simulink model "formation_control"  (R2021a)
settings: Solver=VariableStepAuto  StartTime=0.0  StopTime=T  RelTol=1e-3
undefined symbols (not defined in the file or in its folder): params
settings Model: Creator=gaeta  LastModifiedBy=18214
settings SolverCC: AlgebraicLoopSolver=TrustRegion
settings DataIOCC: InitialState=initialCondition  LoadInitialState=on
settings DebuggingCC: SFMachineParentedDataDiag=warning

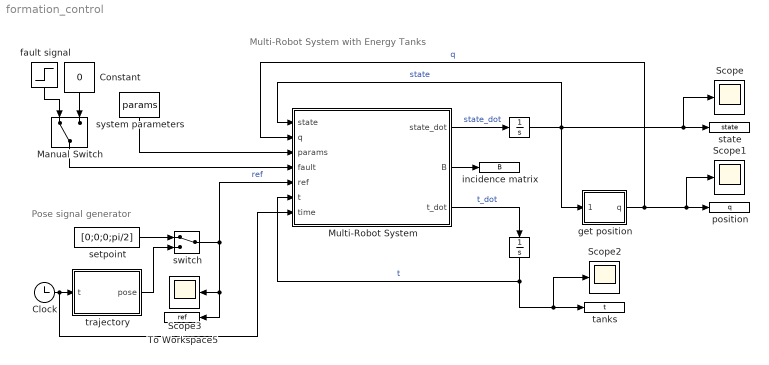
== system formation_control ==
  note: Multi-Robot System with Energy Tanks
  note: Pose signal generator
  "  " : Integrator
  "   " : Integrator
  Clock : Clock
  Constant : Constant  Value=0
  Manual Switch : ManualSwitch
  Multi-Robot System : MATLAB Function  TreatAsAtomicUnit=on
  Scope{,1..3} (4 alike) : Scope
  To Workspace5 : ToWorkspace  VariableName=ref  SaveFormat=Timeseries  SampleTime=-1
  fault signal : Step  Time=25  SampleTime=0
  get position : Subsystem
  incidence matrix : ToWorkspace  VariableName=B  SaveFormat=Timeseries  SampleTime=-1
  position : ToWorkspace  VariableName=q  SaveFormat=Timeseries  SampleTime=-1
  setpoint : Constant  Value=[0;0;0;pi/2]
  state : ToWorkspace  VariableName=state  SaveFormat=Timeseries  SampleTime=-1
  switch : ManualSwitch
  "system parameters " : Constant  Value=params  OutDataTypeStr=Bus: params_bus
  tanks : ToWorkspace  VariableName=t  SaveFormat=Timeseries  SampleTime=-1
  trajectory : MATLAB Function  TreatAsAtomicUnit=on
  wires:
  trajectory/1(pose) -> switch/2
  setpoint/1 -> switch/1
  Clock/1 -> Multi-Robot System/7(time), trajectory/1(t)
  switch/1 -> Multi-Robot System/5(ref), Scope3/1, To Workspace5/1  "ref"
  "system parameters "/1 -> Multi-Robot System/3(params)
  fault signal/1 -> Manual Switch/1
  "  "/1 -> tanks/1, Scope2/1, Multi-Robot System/6(t)  "t"
  Multi-Robot System/1(state_dot) -> "   "/1  "state_dot"
  Multi-Robot System/2(B) -> incidence matrix/1
  "   "/1 -> Multi-Robot System/1(state), Scope/1, state/1, get position/1(state)  "state"
  Multi-Robot System/3(t_dot) -> "  "/1  "t_dot"
  get position/1(q) -> Scope1/1, position/1, Multi-Robot System/2(q)  "q"
  Manual Switch/1 -> Multi-Robot System/4(fault)
  Constant/1 -> Manual Switch/2

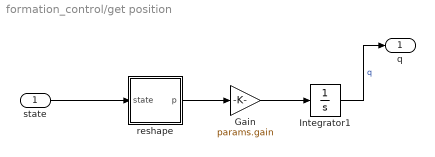
== system formation_control/get position ==
  state : Inport
  Gain : Gain  Gain=params.gain
  Integrator1 : Integrator
  reshape : MATLAB Function  TreatAsAtomicUnit=on
  q : Outport
  wires:
  state/1 -> reshape/1(state)
  reshape/1(p) -> Gain/1
  Gain/1 -> Integrator1/1
  Integrator1/1 -> q/1  "q"

== matlab function formation_control/trajectory ==
  data: pose output size=4; t input size=1
%% 生成参考轨迹
function pose = trajectory(t)
t1 = 5;
t_fault = 25;
t_end = 55;
pause = 5;

w = 0.25;
phi = -w*t1;
A = 80;
z_vel = 1;

y = [0;0;0];
theta = pi/2;
if(t>=t1 && t<t_fault)
    y = [A*sin(w*t+phi); -A*cos(w*t+phi); z_vel*t] - [A*sin(w*t1+phi); -A*cos(w*t1+phi); z_vel*t1];
    theta = atan2(A*sin(w*t+phi), A*cos(w*t+phi));
elseif(t>=t_fault && t<t_fault+pause)
    y = [A*sin(w*t_fault+phi); -A*cos(w*t_fault+phi); z_vel*t_fault] - [A*sin(w*t1+phi); -A*cos(w*t1+phi); z_vel*t1];
    theta = atan2(A*sin(w*t_fault+phi), A*cos(w*t_fault+phi));
elseif(t>=t_fault+pause && t<t_end)
%     y = [A*sin(w*(t-pause)+phi); -A*cos(w*(t-pause)+phi); z_vel*(t-pause)] - [A*sin(w*t1+phi); -A*cos(w*t1+phi); z_vel*t1];
%     theta = atan2(A*sin(w*(t-pause)+phi), A*cos(w*(t-pause)+phi));
    y = [A*sin(w*(t_fault)+phi)+20*w*(t-t_fault-pause); -A*cos(w*(t_fault)+phi)-20*w*(t-t_fault-pause); z_vel*(t_fault)] - [A*sin(w*t1+phi); -A*cos(w*t1+phi); z_vel*t1];
    theta = -pi/4;
elseif(t>=t_end)
%     y = [A*sin(w*(t_end-pause)+phi); -A*cos(w*(t_end-pause)+phi); z_vel*(t_end-pause)] - [A*sin(w*t1+phi); -A*cos(w*t1+phi); z_vel*t1];
%     theta = atan2(A*sin(w*(t_end-pause)+phi), A*cos(w*(t_end-pause)+phi));
    y = [A*sin(w*(t_fault)+phi)+20*w*(t_end-t_fault-pause); -A*cos(w*(t_fault)+phi)-20*w*(t_end-t_fault-pause); z_vel*(t_fault)] - [A*sin(w*t1+phi); -A*cos(w*t1+phi); z_vel*t1];
    theta = -pi/4;
end

pose = [y; theta];
end

== matlab function formation_control/Multi-Robot System ==
  data: state input size=3*(params.N+params.E); q input size=3*params.N; state_dot output size=3*(params.N+params.E); params input; fault input; ref input size=4; t input size=params.N; B output; t_dot output size=params.N; time input
function [state_dot,B,t_dot] = closedLoopSystem(state, q, params, fault, ref, t, time)    % 状态变量（动量、相对位置）、位置、params、失效信号、参考轨迹、能量罐参数（导数）
n = 3;                      % 任务空间
N = params.N;               % Agent数量
faulted_robot = params.faulted_robot;   % 失效Agent

%% 矩阵初始化Ⅰ
p = state(1:n*N);           % Agent动量（状态变量）
m = params.m;               % Agent质量
M = zeros(n*N, n*N);      	% 惯性矩阵
d = params.d;               % 摩擦系数
D = zeros(n*N, n*N);        % 系统（能量）耗散矩阵
for i = 1:N
    M(n*i-n+1:n*i, n*i-n+1:n*i) = eye(n).*m(i);
    D(n*i-n+1:n*i, n*i-n+1:n*i) = eye(n).*d(i);
end

E = params.E;               % 边数

%% 检查失效信号
joined_e = 0;
if(sum(fault)~=0 && ~params.fault_occurred)
    params.fault_occurred = 1;  % 存在失效并更新入度矩阵和失效Agent
    [params.B, joined_e] = faultHandler(params.B, params.Bfull, faulted_robot);
end

%% 矩阵初始化Ⅱ
t_change = 25;
B = params.B;   % B更新
Bcl = kron(params.B,eye(n));	% 克罗内克积求解闭环入度矩阵

dc = params.dc;             % 编队的耗散
Dc = zeros(n*E, n*E);       % 控制器耗散
kc = params.kc;             % 弹簧常数
Kc = zeros(n*E, n*E);       % 弹簧常数矩阵
R = zeros(n*E, n*E);        % n*E matrix containing E rotation matrices

for j = 1:E
    Dc(n*j-n+1:n*j, n*j-n+1:n*j) = eye(n).*dc(j);
    Kc(n*j-n+1:n*j, n*j-n+1:n*j) = eye(n).*kc(j);
    R(n*j-n+1:n*j, n*j-n+1:n*j) = rotz(rad2deg(ref(4)-pi/2));
end

z = state(n*N+1:n*(N+E));	% 相对位置（实际边）
if time <= t_change
    z_des = R*params.z_des1;     % 目标边
else
    z_des = R*params.z_des2;     % 目标边
end

% NOTE: constant matrices M, D, Dc, Kc should be moved in the Init file

%% 能量转移协议
t_dot = zeros(size(t));     % 能量罐参数
w = zeros(E*n,1);           % 转移能量的额外输入

if(params.fault_occurred) 
    Fa_ij = zeros(n,1);
    for i = 1:n
        Fa_ij(i) = Vdot( z(joined_e*n-n+i)-z_des(joined_e*n-n+i) ); % i、j之间相互作用力
    end
    
    i = find(B(:,joined_e)==-1);
    j = find(B(:,joined_e)==1);
    
    Diss = p.'*(inv(M).'*D*inv(M))*p;       % 能量耗散
    
    % 更新i的能量罐和能量罐参数
    wt_ij = -params.gamma(joined_e)*(Fa_ij.'*Fa_ij)*t(i);
    t_dot_i = Diss/t(i) + wt_ij;
    if( all(t(i)>params.tank_max & t_dot_i>0) || all(t(i)<params.tank_min & t_dot_i<0) )
        t_dot(i) = 0;
    else
        t_dot(i) = t_dot_i;
    end
    
    % 更新j的能量罐和能量罐参数
    wt_ji = -params.gamma(joined_e)*(Fa_ij.'*Fa_ij)*t(j);
    t_dot_j = Diss/t(j) + wt_ji;
    if( all(t(j)>params.tank_max & t_dot_j>0) || all(t(j)<params.tank_min & t_dot_j<0) )
        t_dot(j) = 0;
    else
        t_dot(j) = t_dot_j;
    end
    
    % 更新w
    wz_ij = -params.gamma(joined_e)*Fa_ij*t(i)^2 - params.gamma(joined_e)*Fa_ij*t(j)^2;
    w(joined_e*n-n+1:joined_e*n) = wz_ij;
end

%% 轨迹跟踪/队形保持调节
tracking = true;    % 用于启用轨迹跟踪
u = zeros(n*N,1);   % 轨迹跟踪/队形保持控制量
if(tracking)
    
    % 领队轨迹跟踪控制
    Kp = 20;
    u(1:n) = Kp*(ref(1:n)-q(1:n));
    
    % 失效Agent控制
    K_pd = 0.4;
    P_action = K_pd*(-q(n*faulted_robot));
	D_action = 2*K_pd*p(n*faulted_robot)/m(faulted_robot);
    u(n*faulted_robot) = params.fault_occurred*(P_action-D_action);
end

%% 多机系统动力学
Fe = -Bcl * Kc*(z-z_des);           % 外力控制
Fa = -(Bcl*Dc*Bcl.')*(M^(-1)*p);    % 内力控制
p_dot = Fa + Fe - D*(M^(-1)*p) + u;
z_dot = Bcl.'*(M^(-1)*p) + w;
state_dot = [p_dot; z_dot]; % 状态更新

end


% %% 编队内势能函数----------------------------------------------------
% function v = V(error)
% if (error<=0)
%     v = error^2;
% elseif(error>=0 && error<5*pi)
%     v = 50*cos(0.2*error-pi)+50;
% else
%     v = 100;
% end
% end

%% 编队内势能微分函数
function vdot = Vdot(error)
if (error<=0)
    vdot = 2*error;   % 太近了
elseif(error>0 && error<5*pi)
    vdot = 10*sin(0.2*error);   %远了一点
else
    vdot = 0;	% 太远了
end
end

%% 脱离/再入编队操作函数
function [B, joined_edge] = faultHandler(B, Bfull, faulted_robot)
% 脱离失效
if(faulted_robot==1)
    disp("leader cannot be faulted by hypothesis");
else
    faulted_edges = getEdges(faulted_robot, B);
    for e = 1:size(B,2)
        if(ismember(e,faulted_edges))
           B(:,e) = zeros(size(B,1),1); 
        end
    end
end

% 再入失效
if(faulted_robot==size(B,1))
    i = faulted_robot-1;
    j = 1;
else
    i = faulted_robot-1;
    j = faulted_robot+1;
end
joined_edge = getEdge(i,j,Bfull);
B(:,joined_edge) = Bfull(:,joined_edge);
end

% 给定两个Agent，求出连接边
function edges = getEdges(robot, B)
edges = find(B(robot,:)~=0);
end

% 给定两个Agent和全入度矩阵，求出连接边或返回0
function edge = getEdge(i, j, B)
edge = 0;
for e = 1:size(B,2)
    if( (B(i,e)==1 && B(j,e)==-1) || (B(i,e)==-1 && B(j,e)==1) )
        edge = e;
        break
    end
end
end

%

== matlab function formation_control/get position/reshape ==
  data: p output size=3*params.N; state input size=3*(params.N+params.E)
function p = reshape(state)
    %n = 3;
    %N = roots([n/2, n/2, -size(state,1)]).'*(roots([n/2, n/2, -size(state,1)])>0);
    N = 5;
    p = state(1:3*5);
end




%
